simulink model "Demo_Glove"  (R2014a)
settings: Solver=FixedStepDiscrete  SolverMode=SingleTasking  StartTime=0.0  StopTime=inf  FixedStep=0.01  RelTol=1e-3
PostLoadFcn:
  | h_RPStest = RPStest;
model workspace (MAT data in the model file):
  gtest = 0
undefined symbols (not defined in the file or in its folder): avert, avert_gaze_dirs_chance, avert_gaze_duration_factor, avert_head_frequency_factor, avert_head_speed, BML, BML1, BML2, bmlsL, bmlsM, bodyBusyFlag, clock, emotion_amount_factor, faceBusyFlag, fileID, GAZE_WIN, gazing, mutual_gaze_duration_factor, P, pose_chanc_factor, pose_chance_factor, pose_change_flag, pose_frequency_factor, pose_lean, pose_lean_flag, pose_selfAdaptor_chance_factor, pose_speed, pr, serial, STATE_BEFORE, STATE_GO, STATE_OVER, STATE_READY, Stateflow
libraries: simulink x23, instrumentlib x6, lib_affectiveChar_behavior x4, realtime_pacer_lib x2, lib_affectiveChar_input x1
(part 3 of 5)

== matlab function Demo_Glove/facialExpr/facialExprGen/matlabFuncIf/makeBmls ==
  data: i input double size=1 [1..]; arrAU input; eAmount input; arrBML output
function arrBML = fcn(i,arrAU,eAmount)
    %#codegen
    coder.extrinsic('sprintf');
    coder.extrinsic('strcat');
    
    %Maryam, 14-10-2015
    %'strcat' dimension 2  maximum size is 453,it was not possible to concat and send all bmls 
    %for one emotion together(used simulink for loop )    
    
    AU=arrAU(i);eA=eAmount(i);   
    c1 = countDigits(AU);c2 = countDigits(eA);

    str1 = sprintf('<?xml version=\"1.0\" ?><act><bml>');
    
    if(max(ceil(log10(abs(AU))),1)==1) %if AU is one-digit
        temp = sprintf('<face type=\"FACS\" side=\"BOTH\" au=\"%1d\"  start=\"0\" ready=\"1\" stroke=\"2\"  relax=\"300\" end=\"400\" amount=\"%0.1f\"/>',AU,eA); 
        temp2=strcat(str1,temp);
        str1=temp2;
    else      
        temp = sprintf('<face type=\"FACS\" side=\"BOTH\" au=\"%2d\" start=\"0\" ready=\"1\" stroke=\"2\"  relax=\"300\" end=\"400\" amount=\"%0.1f\"/>',AU,eA);
        temp2=strcat(str1,temp);
        str1=temp2;
    end

    str2 = sprintf('</bml></act>');
    %n=length(arrAU);
    %mystr=blanks(arrAU(n));
    mystr=blanks(142+c1+c2);
    mystr = strcat (str1,str2);    
    arrBML = encStr2Arr(mystr);

== stateflow chart Demo_Glove/GazeFollowSubsystem/resetGazeTarget/createGazePawn ==
  state sendSBM(In2) [function]
  state stateCreatePawn
    entry:
    sendSBM(encStr2Arr('scene.getPawn(\"gazeTarget\").setPosition(SrVec(0,1.6,10))'));
  (default) -> stateCreatePawn
  data: In2 function_input double size=[1000 1]

== matlab function Demo_Glove/chack_E_Change1/checkNeutral ==
  data: notNeutral output double size=1; e input
function notNeutral = fcn(e)
%#codegen

if(e~=6)
    notNeutral=1;
else
    notNeutral=0;
end

== matlab function Demo_Glove/EmotionSubsystem/calculateValenceArousal/HEHN_VA_Emo ==
  data: V input; e output double size=1; A input double
function e = fcn(V, A)

aVarTruthTableCondition_1 = false;
aVarTruthTableCondition_2 = false;
aVarTruthTableCondition_3 = false;
aVarTruthTableCondition_4 = false;
aVarTruthTableCondition_5 = false;
aVarTruthTableCondition_6 = false;
aVarTruthTableCondition_7 = false;
aVarTruthTableCondition_8 = false;


% 7-happy  2,1

aVarTruthTableCondition_1 = logical(V>10 && A<10 && A>0);

% 8-ex  1,2 AND 2,2

aVarTruthTableCondition_2 = logical(V>0 && A>10);

% 4-fear  -1,2 AND -2,2

aVarTruthTableCondition_3 = logical(V<0 && A>10);

% 3-frust  -2,1

aVarTruthTableCondition_4 = logical(V<-10 && A<10 && A>0);

% 6-idle  2,-1

aVarTruthTableCondition_5 = logical(V>10 && A<0 && A>-10);

% 5-calm  1,-2 AND 2,-2

aVarTruthTableCondition_6 = logical(V>0 && A<-10);

% 1-bored  -1,-2 AND -2,-2

aVarTruthTableCondition_7 = logical(V<0 && A<-10);

% 2-sad  -2,-1

aVarTruthTableCondition_8 = logical(V<-10 && A<0 && A>-10);

if (aVarTruthTableCondition_1)
    aFcnTruthTableAction_1();
elseif (aVarTruthTableCondition_2)
    aFcnTruthTableAction_2();
elseif (aVarTruthTableCondition_3)
    aFcnTruthTableAction_3();
elseif (aVarTruthTableCondition_4)
    aFcnTruthTableAction_4();
elseif (aVarTruthTableCondition_5)
    aFcnTruthTableAction_5();
elseif (aVarTruthTableCondition_6)
    aFcnTruthTableAction_6();
elseif (aVarTruthTableCondition_7)
    aFcnTruthTableAction_7();
elseif (aVarTruthTableCondition_8)
    aFcnTruthTableAction_8();
else % Default
    aFcnTruthTableAction_5();
end

function aFcnTruthTableAction_1()

% happy

e=7;

function aFcnTruthTableAction_2()

% excited

e=8;

function aFcnTruthTableAction_3()

% fear

e=4;

function aFcnTruthTableAction_4()

% frustration

e=3;

function aFcnTruthTableAction_5()

% idle

e=6;

function aFcnTruthTableAction_6()

% contempt

e=5;

function aFcnTruthTableAction_7()

% bored

e=1;

function aFcnTruthTableAction_8()

% sad

e=2;

== matlab function Demo_Glove/gazeInputArray/makeGazeArray ==
  data: r1 input; y output double size=[1,6]; r2 input; r3 input; r4 input; r5 input; r6 input
function y = fcn(r1,r2,r3,r4,r5,r6)
%#codegen
y=[0,0,0,0,0,0];
y(:,1) = floor(r1);
y(:,2) = floor(r2);
y(:,3) = floor(r3);
y(:,4) = floor(r4);
y(:,5) = floor(r5);
y(:,6) = floor(r6);

== matlab function Demo_Glove/EmotionSubsystem/calculateValenceArousal/LELN_VA_Emo ==
  data: V input; e output double size=1; A input double
function e = fcn(V, A)

aVarTruthTableCondition_1 = false;
aVarTruthTableCondition_2 = false;
aVarTruthTableCondition_3 = false;
aVarTruthTableCondition_4 = false;
aVarTruthTableCondition_5 = false;
aVarTruthTableCondition_6 = false;
aVarTruthTableCondition_7 = false;
aVarTruthTableCondition_8 = false;


% 7-happy  2,1

aVarTruthTableCondition_1 = logical(V>15 && A<15 && A>0);

% 8-ex  1,2 AND 2,2

aVarTruthTableCondition_2 = logical(V>0 && A>15);

% 4-fear  -1,2 AND -2,2

aVarTruthTableCondition_3 = logical(V<0 && A>15);

% 3-frust  -2,1

aVarTruthTableCondition_4 = logical(V<-15 && A<15 && A>0);

% 6-idle  2,-1

aVarTruthTableCondition_5 = logical(V>15 && A<0 && A>-15);

% 5-calm  1,-2 AND 2,-2

aVarTruthTableCondition_6 = logical(V>0 && A<-15);

% 1-bored  -1,-2 AND -2,-2

aVarTruthTableCondition_7 = logical(V<0 && A<-15);

% 2-sad  -2,-1

aVarTruthTableCondition_8 = logical(V<-15 && A<0 && A>-15);

if (aVarTruthTableCondition_1)
    aFcnTruthTableAction_1();
elseif (aVarTruthTableCondition_2)
    aFcnTruthTableAction_2();
elseif (aVarTruthTableCondition_3)
    aFcnTruthTableAction_3();
elseif (aVarTruthTableCondition_4)
    aFcnTruthTableAction_4();
elseif (aVarTruthTableCondition_5)
    aFcnTruthTableAction_5();
elseif (aVarTruthTableCondition_6)
    aFcnTruthTableAction_6();
elseif (aVarTruthTableCondition_7)
    aFcnTruthTableAction_7();
elseif (aVarTruthTableCondition_8)
    aFcnTruthTableAction_8();
else % Default
    aFcnTruthTableAction_5();
end

function aFcnTruthTableAction_1()

% happy

e=7;

function aFcnTruthTableAction_2()

% excited

e=8;

function aFcnTruthTableAction_3()

% fear

e=4;

function aFcnTruthTableAction_4()

% frustration

e=3;

function aFcnTruthTableAction_5()

% idle

e=6;

function aFcnTruthTableAction_6()

% contempt

e=5;

function aFcnTruthTableAction_7()

% bored

e=1;

function aFcnTruthTableAction_8()

% sad

e=2;

== stateflow chart Demo_Glove/CharacterControl/custom_Behavior_Factors ==
  state setP
    entry:
    [mutual_gaze_duration_factor, avert_gaze_duration_factor,avert_head_frequency_factor,avert_head_speed,avert_gaze_dirs_chance]=sharedFunc.setGazeFactors(inV,inA,personality,personalityFlag,vaFlag,gazeArray)
  state init
    entry: mutual_gaze_duration_factor=1;avert_gaze_duration_factor=1;
    avert_head_frequency_factor=1;avert_head_speed=1;avert_gaze_dirs_chance=1;
  state wait
  state setP1
    entry:
    [pose_frequency_factor,pose_chanc_factor,pose_selfAdaptor_chance_factor,pose_lean,pose_speed,pose_lean_flag]=sharedFunc.setPoseFactors(inV,inA,personality,personalityFlag,vaFlag,poseArray,personalityChange)
  state sharedFunc [group]
  (default) -> init
  init -> wait
  setP -> wait
  wait -> setP [order 1] : [gazeArray(:,1)==1]
  setP1 -> wait
  wait -> setP1 [order 2] : [poseArray(:,1)==1]
  data: inA input double size=1; inV input double size=1; vaFlag input boolean size=1; personalityFlag input boolean size=1; gazeArray input double size=[1, 6]; personality input double size=1; personalityChange input boolean size=1; mutual_gaze_duration_factor data_store_memory; avert_head_frequency_factor data_store_memory; avert_gaze_duration_factor data_store_memory; avert_head_speed data_store_memory; avert_gaze_dirs_chance data_store_memory; poseArray input double size=[1, 6]; pose_lean data_store_memory; pose_speed data_store_memory; pose_chanc_factor data_store_memory; pose_frequency_factor data_store_memory; pose_selfAdaptor_chance_factor data_store_memory; pose_lean_flag data_store_memory; emotion_amount_custom input double size=1; emotion_amount_factor data_store_memory size=1

== system Demo_Glove/facialExpr/facialExprGen/emotionBMLsLoop ==
  Amounts : Inport
  AUs : Inport  Port=2
  i : Inport  Port=3  OutMin=1  OutDataTypeStr=double
  e : Inport  Port=4
  Delay : Delay  DelayLength=10  InitialCondition=10
  For Iterator : ForIterator  IterationSource=external
  bml1 : M-S-Function  FunctionName=yarpSendText2_sfun  Parameters='/sim/out/bml9', '/SB/in/bml'
  displayBMLs : MATLAB Function  TreatAsAtomicUnit=on
  loopInBmls : MATLAB Function  TreatAsAtomicUnit=on
  wires:
  AUs/1 -> loopInBmls/2(arrAU)
  Amounts/1 -> loopInBmls/3(eAmount)
  loopInBmls/1(arrBML) -> Delay/1, displayBMLs/3(bml)
  e/1 -> displayBMLs/1(e)
  Delay/1 -> bml1/1
  i/1 -> loopInBmls/1(i), displayBMLs/2(i)

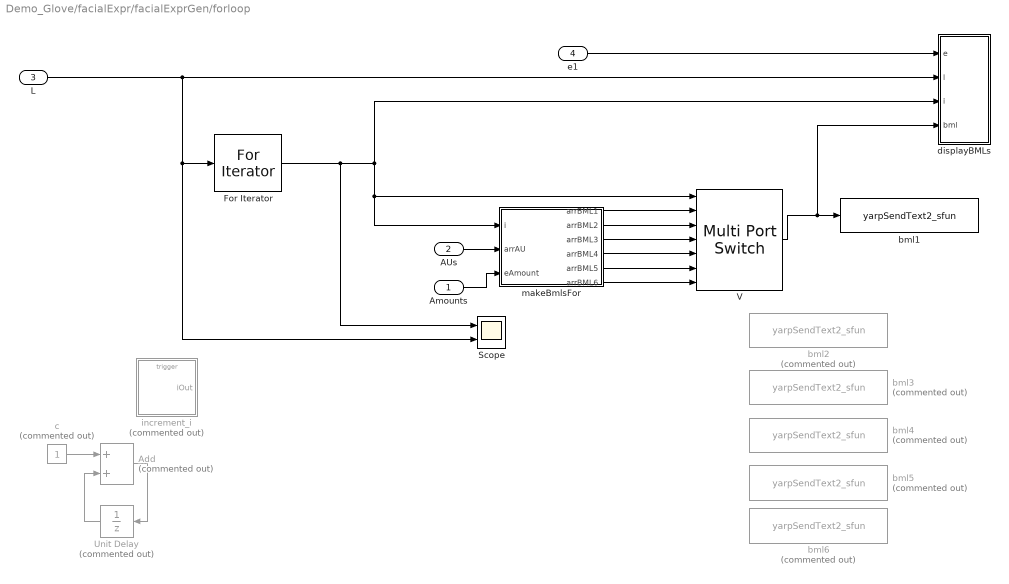
== system Demo_Glove/facialExpr/facialExprGen/forloop ==
  Amounts : Inport
  AUs : Inport  Port=2
  L : Inport  Port=3
  e1 : Inport  Port=4
  Add : Sum  Commented=on
  For Iterator : ForIterator  IterationSource=external  IterationVariableDataType=double
  Scope : Scope  NumInputPorts=2
      settings: YMin=3~3  YMax=3~3  SaveName=ScopeData7
  Unit Delay : UnitDelay  Commented=on  SampleTime=0.01
  V : MultiPortSwitch  Inputs=6
  bml1 : M-S-Function  FunctionName=yarpSendText2_sfun  Parameters='/sim/out/bml9', '/SB/in/bml'
  bml2 : M-S-Function  Commented=on  FunctionName=yarpSendText2_sfun  Parameters='/sim/out/bml10', '/SB/in/bml'
  bml3 : M-S-Function  Commented=on  FunctionName=yarpSendText2_sfun  Parameters='/sim/out/bml11', '/SB/in/bml'
  bml4 : M-S-Function  Commented=on  FunctionName=yarpSendText2_sfun  Parameters='/sim/out/bml12', '/SB/in/bml'
  bml5 : M-S-Function  Commented=on  FunctionName=yarpSendText2_sfun  Parameters='/sim/out/bml13', '/SB/in/bml'
  bml6 : M-S-Function  Commented=on  FunctionName=yarpSendText2_sfun  Parameters='/sim/out/bml14', '/SB/in/bml'
  c : Constant  Commented=on
  displayBMLs : MATLAB Function  TreatAsAtomicUnit=on
  increment_i : Subsystem  Commented=on
  makeBmlsFor : MATLAB Function  TreatAsAtomicUnit=on
  wires:
  L/1 -> Scope/2, For Iterator/1, displayBMLs/2(l)
  AUs/1 -> makeBmlsFor/2(arrAU)
  Amounts/1 -> makeBmlsFor/3(eAmount)
  e1/1 -> displayBMLs/1(e)
  Unit Delay/1 -> Add/2
  c/1 -> Add/1
  Add/1 -> Unit Delay/1
  For Iterator/1 -> Scope/1, V/1, makeBmlsFor/1(i), displayBMLs/3(i)
  V/1 -> displayBMLs/4(bml), bml1/1
  makeBmlsFor/1(arrBML1) -> V/2
  makeBmlsFor/2(arrBML2) -> V/3
  makeBmlsFor/3(arrBML3) -> V/4
  makeBmlsFor/4(arrBML4) -> V/5
  makeBmlsFor/5(arrBML5) -> V/6
  makeBmlsFor/6(arrBML6) -> V/7

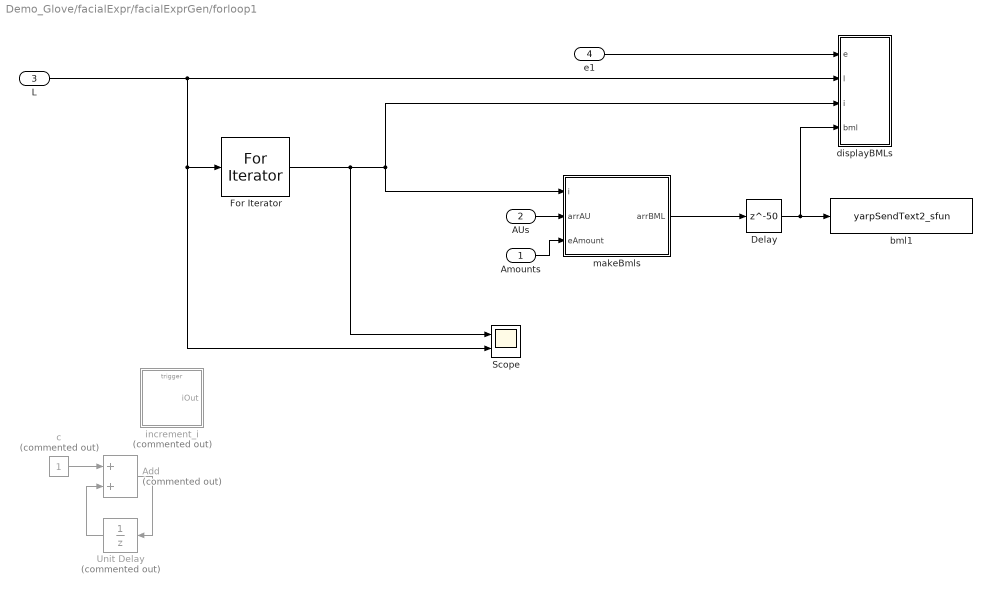
== system Demo_Glove/facialExpr/facialExprGen/forloop1 ==
  Amounts : Inport
  AUs : Inport  Port=2
  L : Inport  Port=3
  e1 : Inport  Port=4
  Add : Sum  Commented=on
  Delay : Delay  DelayLength=50  InitialCondition=0
  For Iterator : ForIterator  IterationSource=external  IterationVariableDataType=double
  Scope : Scope  NumInputPorts=2
      settings: YMin=3~3  YMax=3~3  SaveName=ScopeData7
  Unit Delay : UnitDelay  Commented=on  SampleTime=0.01
  bml1 : M-S-Function  FunctionName=yarpSendText2_sfun  Parameters='/sim/out/bml9', '/SB/in/bml'
  c : Constant  Commented=on
  displayBMLs : MATLAB Function  TreatAsAtomicUnit=on
  increment_i : Subsystem  Commented=on
  makeBmls : MATLAB Function  TreatAsAtomicUnit=on
  wires:
  L/1 -> Scope/2, For Iterator/1, displayBMLs/2(l)
  AUs/1 -> makeBmls/2(arrAU)
  Amounts/1 -> makeBmls/3(eAmount)
  e1/1 -> displayBMLs/1(e)
  makeBmls/1(arrBML) -> Delay/1
  Unit Delay/1 -> Add/2
  c/1 -> Add/1
  Add/1 -> Unit Delay/1
  For Iterator/1 -> Scope/1, makeBmls/1(i), displayBMLs/3(i)
  Delay/1 -> displayBMLs/4(bml), bml1/1

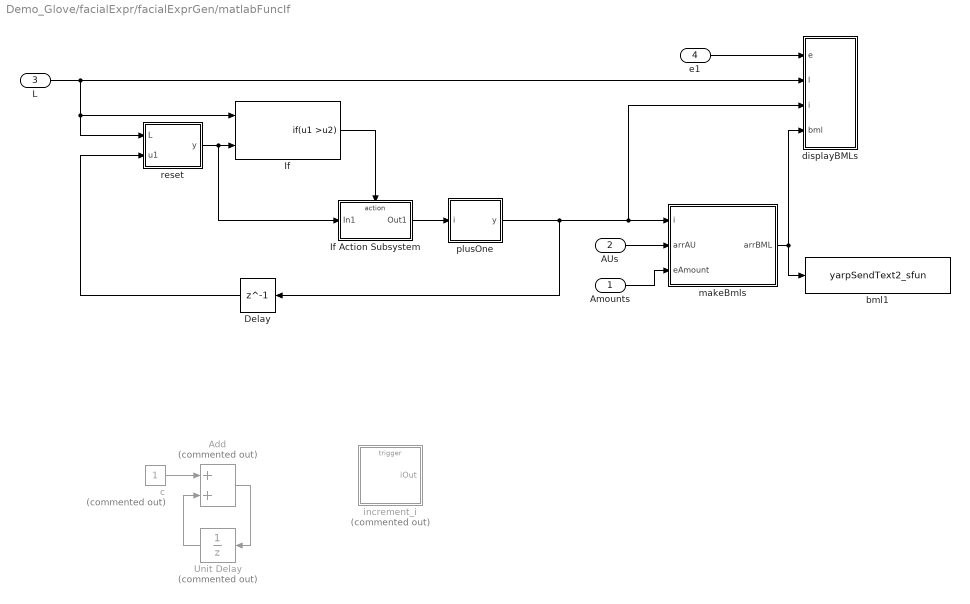
== system Demo_Glove/facialExpr/facialExprGen/matlabFuncIf ==
  Amounts : Inport
  AUs : Inport  Port=2
  L : Inport  Port=3
  e1 : Inport  Port=4
  Add : Sum  Commented=on
  Delay : Delay  DelayLength=1  InitialCondition=0
  If : If  NumInputs=2  IfExpression=u1 >u2  ShowElse=off
  If Action Subsystem : Subsystem  TreatAsAtomicUnit=on
  Unit Delay : UnitDelay  Commented=on  SampleTime=0.01
  bml1 : M-S-Function  FunctionName=yarpSendText2_sfun  Parameters='/sim/out/bml9', '/SB/in/bml'
  c : Constant  Commented=on
  displayBMLs : MATLAB Function  TreatAsAtomicUnit=on
  increment_i : Subsystem  Commented=on
  makeBmls : MATLAB Function  TreatAsAtomicUnit=on
  plusOne : MATLAB Function  TreatAsAtomicUnit=on
  reset : MATLAB Function  TreatAsAtomicUnit=on
  wires:
  L/1 -> reset/1(L), If/1, displayBMLs/2(l)
  AUs/1 -> makeBmls/2(arrAU)
  Amounts/1 -> makeBmls/3(eAmount)
  e1/1 -> displayBMLs/1(e)
  makeBmls/1(arrBML) -> displayBMLs/4(bml), bml1/1
  plusOne/1(y) -> Delay/1, displayBMLs/3(i), makeBmls/1(i)
  If/1 -> If Action Subsystem/Action
  Unit Delay/1 -> Add/2
  c/1 -> Add/1
  Add/1 -> Unit Delay/1
  If Action Subsystem/1(Out1) -> plusOne/1(i)
  Delay/1 -> reset/2(u1)
  reset/1(y) -> If Action Subsystem/1(In1), If/2

== system Demo_Glove/readGlove/normal glove/Normalize Index ==
  RawGlove : Inport
  Divide : Product  Inputs=*/  OutDataTypeStr=double  RndMeth=Nearest  InputSameDT=on
  Divide1 : Product  Inputs=**
  MinMax : Subsystem
  Range : Sum  Inputs=+-  OutDataTypeStr=double
  Ring1 : Constant  Value=100
  Subtract5 : Sum  Inputs=+-  OutDataTypeStr=double
  Norm100Out : Outport
  wires:
  MinMax/2(Max) -> Range/1
  Ring1/1 -> Divide1/2
  Subtract5/1 -> Divide/1
  MinMax/1(Min) -> Subtract5/2, Range/2
  RawGlove/1 -> Subtract5/1, MinMax/1(In1)
  Divide1/1 -> Norm100Out/1
  Divide/1 -> Divide1/1
  Range/1 -> Divide/2

== system Demo_Glove/readGlove/normal glove/Normalize Middle ==
  RawGlove : Inport
  Divide : Product  Inputs=*/  OutDataTypeStr=double  RndMeth=Nearest  InputSameDT=on
  Divide1 : Product  Inputs=**
  MinMax : Subsystem
  Range : Sum  Inputs=+-  OutDataTypeStr=double
  Ring1 : Constant  Value=100
  Subtract5 : Sum  Inputs=+-  OutDataTypeStr=double
  Norm100Out : Outport
  wires:
  MinMax/2(Max) -> Range/1
  Ring1/1 -> Divide1/2
  Subtract5/1 -> Divide/1
  MinMax/1(Min) -> Subtract5/2, Range/2
  RawGlove/1 -> Subtract5/1, MinMax/1(In1)
  Divide1/1 -> Norm100Out/1
  Divide/1 -> Divide1/1
  Range/1 -> Divide/2

== system Demo_Glove/readGlove/normal glove/Normalize Ring ==
  RawGlove : Inport
  Divide : Product  Inputs=*/  OutDataTypeStr=double  RndMeth=Nearest  InputSameDT=on
  Divide1 : Product  Inputs=**
  MinMax : Subsystem
  Range : Sum  Inputs=+-  OutDataTypeStr=double
  Ring1 : Constant  Value=100
  Subtract5 : Sum  Inputs=+-  OutDataTypeStr=double
  Norm100Out : Outport
  wires:
  MinMax/2(Max) -> Range/1
  Ring1/1 -> Divide1/2
  Subtract5/1 -> Divide/1
  MinMax/1(Min) -> Subtract5/2, Range/2
  RawGlove/1 -> Subtract5/1, MinMax/1(In1)
  Divide1/1 -> Norm100Out/1
  Divide/1 -> Divide1/1
  Range/1 -> Divide/2

== system Demo_Glove/facialExpr/facialExprGen/forloop/increment_i ==
  Trigger : TriggerPort  PortDimensions=1
  Add : Sum
  Scope : Scope  NumInputPorts=2
      settings: TimeRange=10  YMin=-5~-5  YMax=5~5  SaveName=ScopeData3
  Unit Delay : UnitDelay  SampleTime=0.01
  c : Constant
  iOut : Outport  OutMin=1  OutDataTypeStr=double  InitialOutput=1
  wires:
  Add/1 -> Scope/1, iOut/1, Unit Delay/1
  Unit Delay/1 -> Scope/2, Add/2
  c/1 -> Add/1

== system Demo_Glove/facialExpr/facialExprGen/forloop1/increment_i ==
  Trigger : TriggerPort  PortDimensions=1
  Add : Sum
  Scope : Scope  NumInputPorts=2
      settings: TimeRange=10  YMin=-5~-5  YMax=5~5  SaveName=ScopeData3
  Unit Delay : UnitDelay  SampleTime=0.01
  c : Constant
  iOut : Outport  OutMin=1  OutDataTypeStr=double  InitialOutput=1
  wires:
  Add/1 -> Scope/1, iOut/1, Unit Delay/1
  Unit Delay/1 -> Scope/2, Add/2
  c/1 -> Add/1

== system Demo_Glove/facialExpr/facialExprGen/matlabFuncIf/If Action Subsystem ==
  In1 : Inport
  Action Port : ActionPort  ActionType=then
  Scope : Scope
      settings: SaveName=ScopeData8
  Out1 : Outport
  wires:
  In1/1 -> Scope/1, Out1/1

== system Demo_Glove/facialExpr/facialExprGen/matlabFuncIf/increment_i ==
  Trigger : TriggerPort  PortDimensions=1
  Add : Sum
  Scope : Scope  NumInputPorts=2
      settings: TimeRange=10  YMin=-5~-5  YMax=5~5  SaveName=ScopeData3
  Unit Delay : UnitDelay  SampleTime=0.01
  c : Constant
  iOut : Outport  OutMin=1  OutDataTypeStr=double  InitialOutput=1
  wires:
  Add/1 -> Scope/1, iOut/1, Unit Delay/1
  Unit Delay/1 -> Scope/2, Add/2
  c/1 -> Add/1

== system Demo_Glove/readGlove/normal glove/Normalize Index/MinMax ==
  In1 : Inport
  Index1 : Constant  Value=0
  MinMax Running Resettable : simulink/Math Operations/MinMax Running Resettable  Function=min  vinit=100
  MinMax Running Resettable1 : simulink/Math Operations/MinMax Running Resettable  Function=max  vinit=0.0
  Min : Outport
  Max : Outport  Port=2
  wires:
  Index1/1 -> MinMax Running Resettable/2, MinMax Running Resettable1/2
  MinMax Running Resettable/1 -> Min/1
  In1/1 -> MinMax Running Resettable/1, MinMax Running Resettable1/1
  MinMax Running Resettable1/1 -> Max/1

== system Demo_Glove/readGlove/normal glove/Normalize Middle/MinMax ==
  In1 : Inport
  Index1 : Constant  Value=0
  MinMax Running Resettable : simulink/Math Operations/MinMax Running Resettable  Function=min  vinit=100
  MinMax Running Resettable1 : simulink/Math Operations/MinMax Running Resettable  Function=max  vinit=0.0
  Min : Outport
  Max : Outport  Port=2
  wires:
  Index1/1 -> MinMax Running Resettable/2, MinMax Running Resettable1/2
  MinMax Running Resettable/1 -> Min/1
  In1/1 -> MinMax Running Resettable/1, MinMax Running Resettable1/1
  MinMax Running Resettable1/1 -> Max/1

== system Demo_Glove/readGlove/normal glove/Normalize Ring/MinMax ==
  In1 : Inport
  Index1 : Constant  Value=0
  MinMax Running Resettable : simulink/Math Operations/MinMax Running Resettable  Function=min  vinit=100
  MinMax Running Resettable1 : simulink/Math Operations/MinMax Running Resettable  Function=max  vinit=0.0
  Min : Outport
  Max : Outport  Port=2
  wires:
  Index1/1 -> MinMax Running Resettable/2, MinMax Running Resettable1/2
  MinMax Running Resettable/1 -> Min/1
  In1/1 -> MinMax Running Resettable/1, MinMax Running Resettable1/1
  MinMax Running Resettable1/1 -> Max/1

== stateflow chart Demo_Glove/CharacterControl ==
  note: High Priority Tasks: Hand gesture for game
  state RPS_Scenario [parallel]
    settings: executionOrder=1
  note: Middle Priority Tasks: wave back at user and distance regulation
  state personalSpace_Controller [parallel]
    settings: executionOrder=5
  state wave_Controller [parallel]
    settings: executionOrder=7
  note: Low Priority Tasks: Idle gaze, pose and facial Expressions:
  state idlePose_Controller [parallel]
    settings: executionOrder=3
  state Gaze_Controller [parallel]
    settings: executionOrder=2
  state facialExpression_Controller [parallel]
    settings: executionOrder=4
  note: Parameters (can change
      | to seethe rangeof results)
      | -mutual_gaze_duration_factor
      | -avert_gaze_duration_factor
      | -avert_head_frequency_factor
      | -avert_head_speed(fast/slow/normal)
      | -avert_gaze_dirs_chance (down/up/normal)
      |
      | Inputs:(needed)
      | -faceAttendingFlag
      | -bodyAttendingFlag
  note: Parameters:
      | pose_selfAdaptor_chance_factor
      | pose_chance_factor
      | pose_frequency_factor
      | pose_speed(fast,slow,normal)
      | pose_lean(forward,backward,normal)
      |
      | Inputs:
      | -bodyAttendingFlag
  note: Parameters:
      |
      | Inputs:
      | -faceAttendingFlag
  note: Internal emotion/personality affects behavior modules (smile, gaze, pose)
  note: Instead of setting the factors directly in behavior or personality-emotion, added a module to centerlized and encapsulate all factors affecting behavior and their weights.
  state personality_Behavior_Factors [parallel]
    settings: executionOrder=9
  state emotion_Behavior_Factors [parallel]
    settings: executionOrder=10
  state custom_Behavior_Factors [parallel]
    settings: executionOrder=11
  note: Attention: if body or face is attending, no idle behavior are generated.
      | A queue is defined to priortize behaviors based on their importance.
  state attention_Controller [parallel]
    settings: executionOrder=8
  state sendBMLbyPriority [parallel]
    settings: executionOrder=6
    state sendH
      entry: BML=bmlsH(:,1);
      sendBML(BML);
      newBmlsH=removeQueue(bmlsH);
      bmlsH=newBmlsH;
    state init
      entry: n=encStr2Arr(' ');
      bmlsH=[n n n n n];
      bmlsM=[n n n n n];
      bmlsL=[n n n n n];
    state checkHighPriority
      entry:
      hEmpty=isEmptyQueue(bmlsH);
    state sendM
      entry: BML=bmlsM(:,1);
      sendBML(BML);
      newBmlsM= removeQueue(bmlsM);
      bmlsM=newBmlsM;
    state Mid
      entry:mEmpty=isEmptyQueue(bmlsM);
    state sendL
      entry: BML=bmlsL(:,1);
      sendBML(BML);
      newBmlsL= removeQueue(bmlsL);
      bmlsL=newBmlsL;
    state low
      entry:
      lEmpty=isEmptyQueue(bmlsL);
    note: Arrows' execution order is very importan here!
    state sendBML(In1) [function]
    sendH -> checkHighPriority
    checkHighPriority -> sendH [order 2] : [hEmpty~=1]
    (default) -> init
    init -> checkHighPriority
    checkHighPriority -> Mid [order 1] : [hEmpty==1]
    Mid -> checkHighPriority [order 4] : [mEmpty==1]
    sendM -> checkHighPriority [order 2]
    sendL -> checkHighPriority [order 3]
    low -> sendH [order 1] : [isEmptyQueue(bmlsH)~=1]
    Mid -> sendH [order 1] : [isEmptyQueue(bmlsH)~=1]
    sendM -> sendH [order 1] : [isEmptyQueue(bmlsH)~=1]
    sendL -> sendH [order 2] : [isEmptyQueue(bmlsH)~=1]
    Mid -> sendM [order 2] : [mEmpty~=1]
    Mid -> low [order 3] : [mEmpty==1]
    low -> Mid [order 4] : [lEmpty==1]
    low -> sendM [order 2] : [isEmptyQueue(bmlsM)~=1]
    sendL -> sendM [order 1] : [isEmptyQueue(bmlsM)~=1]
    low -> sendL [order 3] : [lEmpty~=1]
  data: In1 function_input double size=[1000 1]; bmls function_input; newBmls function_output; bmls function_input; empty function_output; emotion_amount_custom input double size=1; randArray input double size=[1,25]; poseArray input double size=[1,6]; gazeArray input double size=[1,6]; gameState output double size=1; inputUser input double size=1; bradHand output double size=1; userHand output double size=1; win output double size=1; temp local double size=1; diff local double size=1; uHand local double size=1; bHand local double size=1; bWinT output double size=1; uWinT output double size=1; randSmile local double size=1; boredom local double size=1; BOREDOM_THRESHOLD local double size=1; randAvertGazeChance local double size=1; randPoseChance local double size=1; interest local double size=1; r local double size=1; pa local double size=1; s local double size=1; randGazeDur local double size=1; P local double size=1 =0; smileN local double size=1; isSmiling input double size=1; body_isAttending input boolean size=1; face_isAttending input boolean size=1; avert local double size=1; GAZE_GUI local double size=1; GAZE_SOFTEYE local double size=1; GAZE_USER_HAND local double size=1; STATE_READY local double size=1 =0; STATE_GO local double size=1 =1; STATE_HAND local double size=1 =2; STATE_OVER local double size=1 =3; gazing local double size=1; GAZE_WIN local double size=1; randSlowPose local double size=1; STATE_BEFORE local double size=1 =4; STATE_RESULT local double size=1 =5; STATE_WAIT local double size=1 =6; HAPPY local double size=1 =4; SAD local double size=1 =4; CONTEMPT local double size=1 =4; BORED local double size=1 =4; FRUST local double size=1 =4; FEAR local double size=1 =4; IDLE local double size=1 =4; EXCITE local double size=1 =4; BML local double size=[1000,1]; pr local double size=1; t1 local; t2 local; round output double size=1; newBmlA local; fileID local double; xChangeFlag input boolean size=1; zChangeFlag input boolean size=1; isInvading input double size=1; inA input double size=1; handUp input double size=1; inV input double size=1; internalE input double size=1; personality input double size=1; BML2 local double size=[1000,1]; BML1 local double size=[1000,1]; t local double size=1; bodyBusyFlag local double size=1; n local double size=[1000,1]; bmlsL local double size=[1000,5]; hEmpty local double size=1; bmlsH local double size=[1000,5]; newBmlsH local double size=[1000,5]; newBmlsL local double size=[1000,5]; lEmpty local; newBmlsM local double size=[1000,5]; bmlsM local double size=[1000,5]; mEmpty local; avertH local double size=1; emoChange input boolean size=1; personalityChange input boolean size=1; faceBusyFlag local double size=1; personalityFlag input boolean size=1; vaFlag input boolean size=1; mutual_gaze_duration_factor local double size=1; avert_gaze_duration_factor local double size=1; avert_head_frequency_factor local double size=1; avert_gaze_dirs_chance local double size=1; avert_head_speed local double size=1; pose_chance_factor local double size=1; pose_selfAdaptor_chance_factor local double size=1; pose_frequency_factor local double size=1; pose_speed local double size=1; pose_lean local double size=1; pose_lean_flag local double size=1; pose_change_flag local double size=1; emotion_amount_factor local double size=[1,6]
  events: secs input RISING_EDGE_EVENT
  function newBmls=removeQueue(bmls):
    | function newBmls=removeQueue(bmls) 
    |     n=encStr2Arr(' ');
    |     newBmls=[n n n n n];
    |     newBmls(:,1)= bmls(:,2);
    |     newBmls(:,2)= bmls(:,3);
    |     newBmls(:,3)= bmls(:,4);
    |     newBmls(:,4)= bmls(:,5);
    |     newBmls(:,5)=encStr2Arr(' ');
  function empty=isEmptyQueue(bmls):
    | function empty=isEmptyQueue(bmls)
    | empty=1;
    | tempp=encStr2Arr(' ');
    | for i = 1:5
    |     if (isequal(bmls(:,i),tempp)==0)%there is a cell which is not equal to null
    |         empty=0;
    |         break
    |     end
    | end

== matlab function Demo_Glove/sendtoGUIFunction ==
  data: gameStatus input; bradHand input; userHand input; win input; bTotal input; uTotal input; gameNum input
function fcn(gameStatus, bradHand,userHand,win,bTotal,uTotal,gameNum)
%#codegen
setappdata(0,'gameStatus',gameStatus) 
setappdata(0,'bradHand',bradHand) 
setappdata(0,'userHand',userHand) 
setappdata(0,'win',win) 
setappdata(0,'uTotal',uTotal) 
setappdata(0,'bTotal',bTotal) 
setappdata(0,'gameNum',gameNum)

== matlab function Demo_Glove/readGlove/convertFunction ==
  data: u input; y output
function y = fcn(u)
%#codegen
%    paper=0; 'rock'=3;'scissors'=1;
%to 'paper'=1;'rock'=2;'scissors'=0;

if(u==0)
    u=1;
elseif(u==1)
    u=0;
elseif(u==3)
    u=2;
else 
    u=3;
end
y = u;
